simulink model "s_position_pv_ip01_2"  (R2025b)
settings: Solver=ode1  StartTime=0.0  StopTime=50  FixedStep=0.001  RelTol=1e-3  AbsTol=1e-6
libraries: simulink x3
settings Model: Creator=MLevis  LastModifiedBy=USER_NAME
settings SolverCC: AutoScaleAbsTol=off  AlgebraicLoopSolver=TrustRegion
settings DataIOCC: SaveFormat=Array  SignalLoggingSaveFormat=ModelDataLogs  ReturnWorkspaceOutputs=off
settings OptimizationCC: BlockReduction=off  BooleanDataType=off  OptimizeBlockIOStorage=off  BufferReuse=off  ExpressionFolding=off  ExpressionDepthLimit=2147483647.0  LocalBlockOutputs=off  InitFltsAndDblsToZero=on  LifeSpan=inf
settings DebuggingCC: SaveWithParameterizedLinksMsg=none  UnderspecifiedInitializationDetection=Classic  MergeDetectMultiDrivingBlocksExec=none  SignalResolutionControl=TryResolveAllWithWarning  MultiTaskDSMMsg=warning  MultiTaskCondExecSysMsg=none  FcnCallInpInsideContextMsg=warning  UnconnectedInputMsg=warning  UnconnectedOutputMsg=warning  UnconnectedLineMsg=warning  StateNameClashWarn=warning  SFUnexpectedBacktrackingDiag=warning  SFNoUnconditionalDefaultTransitionDiag=warning  SFExecutionAtInitializationDiag=none  ArithmeticOperatorsInVariantConditions=warning
settings HardwareCC: ProdBitPerPointer=32.0  ProdBitPerSizeT=32.0  ProdBitPerPtrDiffT=32.0  ProdLargestAtomicFloat=None  ProdIntDivRoundTo=Undefined  ProdEndianess=Unspecified  ProdWordSize=32.0  ProdHWDeviceType=32-bit Generic  TargetUnknown=on
settings ModelReferenceCC: PropagateSignalLabelsOutOfModel=off
settings RTWCC: SystemTargetFile=wincon.tlc  MakeCommand=make_wc  TemplateMakefile=nt_msvc.tmf  GPUComputeCapability=3.5
settings CodeAppCC: StateflowObjectComments=on
settings STFCustomTargetCC: SystemTargetFile=wincon.tlc  TargetFcnLib=ansi_tfl_tmw.mat  ModelReferenceCompliant=off  ConcurrentExecutionCompliant=off  MATLABClassNameForMDSCustomization=Simulink.SoftwareTarget.TargetSpecificTriggerConfigurationBase
settings ConfigComp: CovMetricSettings=dw  CovSaveCumulativeToWorkspaceVar=on  CovSaveSingleToWorkspaceVar=on

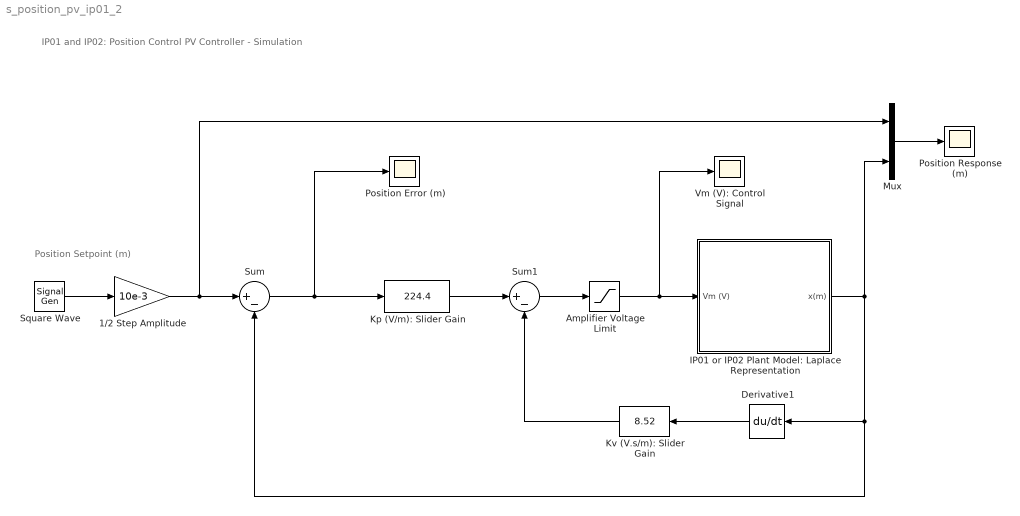
== system s_position_pv_ip01_2 ==
  note: Position Setpoint (m)
  note: IP01 and IP02: Position Control
      | PV Controller - Simulation
  1/2 Step Amplitude : Gain  Gain=10e-3  SaturateOnIntegerOverflow=on  OutDataTypeStr=Inherit: Same as input  ParamDataTypeStr=Inherit: Same as input
  Amplifier Voltage Limit : Saturate  UpperLimit=24  LowerLimit=- 24
  Derivative1 : Derivative  CoefficientInTFapproximation=0.955
  IP01 or IP02 Plant Model: Laplace Representation : Subsystem
  Kp (V/m): Slider Gain : simulink/Math Operations/Slider Gain  gain=224.4  low=0  high=700
  Kv (V.s/m): Slider Gain : simulink/Math Operations/Slider Gain  gain=8.52  low=0  high=40
  Mux : Mux  Inputs=2
  Position Response (m) : Scope
      settings: SampleTime=0.001  TimeSpan=5  ActiveDisplayYMinimum=-0.02  ActiveDisplayYMaximum=0.02  DataLoggingVariableName=ScopeData4  DataLoggingSaveFormat=Array
  Position Error (m) : Scope
      settings: SampleTime=0.001  TimeSpan=2  ActiveDisplayYMinimum=-0.02  ActiveDisplayYMaximum=0.02  DataLoggingSaveFormat=Array
  Square Wave : SignalGenerator  WaveForm=square  Frequency=0.66
  Sum : Sum  Inputs=|+-  InputSameDT=on  SaturateOnIntegerOverflow=on  OutDataTypeStr=Inherit: Same as first input
  Sum1 : Sum  Inputs=|+-  InputSameDT=on  SaturateOnIntegerOverflow=on  OutDataTypeStr=Inherit: Same as first input
  Vm (V): Control Signal : Scope
      settings: SampleTime=0.001  TimeSpan=5  ActiveDisplayYMinimum=-15  ActiveDisplayYMaximum=15  DataLoggingVariableName=ScopeData5  DataLoggingSaveFormat=Array
  wires:
  Sum/1 -> Kp (V/m): Slider Gain/1, Position Error (m)/1
  Sum1/1 -> Amplifier Voltage Limit/1
  1/2 Step Amplitude/1 -> Sum/1, Mux/1
  IP01 or IP02 Plant Model: Laplace Representation/1(x(m)) -> Sum/2, Derivative1/1, Mux/2
  Derivative1/1 -> Kv (V.s/m): Slider Gain/1
  Mux/1 -> Position Response (m)/1
  Square Wave/1 -> 1/2 Step Amplitude/1
  Kp (V/m): Slider Gain/1 -> Sum1/1
  Kv (V.s/m): Slider Gain/1 -> Sum1/2
  Amplifier Voltage Limit/1 -> IP01 or IP02 Plant Model: Laplace Representation/1(Vm (V)), Vm (V): Control Signal/1

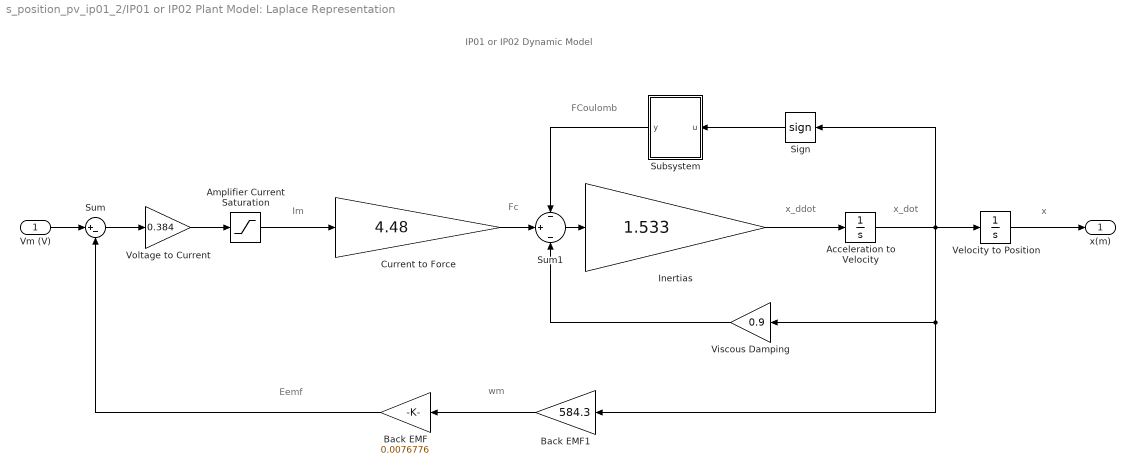
== system s_position_pv_ip01_2/IP01 or IP02 Plant Model: Laplace Representation ==
  note: FCoulomb
  note: IP01 or IP02 Dynamic Model
  note: Fc
  note: Im
  note: Eemf
  note: wm
  note: x_dot
  note: x_ddot
  note: x
  Vm (V) : Inport
  Acceleration to Velocity : Integrator
  Amplifier Current Saturation : Saturate  UpperLimit=4  LowerLimit=-4
  Back EMF : Gain  Gain=0.0076776  SaturateOnIntegerOverflow=on  OutDataTypeStr=Inherit: Same as input  ParamDataTypeStr=Inherit: Same as input
  Back EMF1 : Gain  Gain=584.3  SaturateOnIntegerOverflow=on  OutDataTypeStr=Inherit: Same as input  ParamDataTypeStr=Inherit: Same as input
  Current to Force : Gain  Gain=4.48  SaturateOnIntegerOverflow=on  OutDataTypeStr=Inherit: Same as input  ParamDataTypeStr=Inherit: Same as input
  Inertias : Gain  Gain=1.533  SaturateOnIntegerOverflow=on  OutDataTypeStr=Inherit: Same as input  ParamDataTypeStr=Inherit: Same as input
  Sign : Signum
  Subsystem : Subsystem
  Sum : Sum  Inputs=|+-  InputSameDT=on  SaturateOnIntegerOverflow=on  OutDataTypeStr=Inherit: Same as first input
  Sum1 : Sum  Inputs=-|+|-  InputSameDT=on  SaturateOnIntegerOverflow=on  OutDataTypeStr=Inherit: Same as first input
  Velocity to Position : Integrator
  Viscous Damping : Gain  Gain=0.9  SaturateOnIntegerOverflow=on  OutDataTypeStr=Inherit: Same as input  ParamDataTypeStr=Inherit: Same as input
  Voltage to Current : Gain  Gain=0.384  SaturateOnIntegerOverflow=on  OutDataTypeStr=Inherit: Same as input  ParamDataTypeStr=Inherit: Same as input
  x(m) : Outport
  wires:
  Sum/1 -> Voltage to Current/1
  Inertias/1 -> Acceleration to Velocity/1
  Sum1/1 -> Inertias/1
  Voltage to Current/1 -> Amplifier Current Saturation/1
  Acceleration to Velocity/1 -> Viscous Damping/1, Back EMF1/1, Velocity to Position/1, Sign/1
  Back EMF1/1 -> Back EMF/1
  Vm (V)/1 -> Sum/1
  Velocity to Position/1 -> x(m)/1
  Current to Force/1 -> Sum1/2
  Viscous Damping/1 -> Sum1/3
  Back EMF/1 -> Sum/2
  Amplifier Current Saturation/1 -> Current to Force/1
  Sign/1 -> Subsystem/1(u)
  Subsystem/1(y) -> Sum1/1

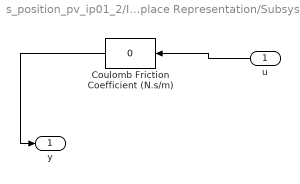
== system s_position_pv_ip01_2/IP01 or IP02 Plant Model: Laplace Representation/Subsystem ==
  u : Inport
  Coulomb Friction Coefficient (N.s/m) : simulink/Math Operations/Slider Gain  gain=0  low=0  high=3
  y : Outport
  wires:
  Coulomb Friction Coefficient (N.s/m)/1 -> y/1
  u/1 -> Coulomb Friction Coefficient (N.s/m)/1
